simulink model "Autopilot_q_full_5may_new"  (R2020a)
settings: Solver=ode4  StartTime=0.0  StopTime=300  FixedStep=0.01  RelTol=1e-3
undefined symbols (not defined in the file or in its folder): Aero_cofficients, Atmosphere_pert, Atmospheric_model, Counter_sensor_model, Earth, error_global, flags_global, Guidance_Flags_global, INT_global, param_guidance, Payload_data, Plane_state_mode_finish_catcher_ftr_mode, Plane_state_mode_finish_catcher_fw_mode, Plane_state_mode_finish_catcher_q_mode, Plane_state_mode_finish_catcher_rtr_mode, Plane_state_store, propulsion_model, propulsion_model_int, Structural_data, Thrust_data_store, time_global, WGS84, Wind_data, Wind_model_int, Wind_pert_factor
libraries: simulink x33, aerolibactuator x15, cstblocks x3, aerolibatmos2 x2, aerolibfltsims x1, aerolibtransform2 x1, shared6dof x1
(part 5 of 10)

== system Autopilot_q_full_5may_new/AUTOPILOT /Autopilot Transition mode/Forward transition/Roll controller ==
  a_y_d : Inport
  In2 : Inport  Port=2
  Aero_coffecients read3 : DataStoreRead  DataStoreName=Aero_cofficients  DataStoreElements=Aero_cofficients(:,:)
  Constant{6..11} (6 alike) : Constant
  Data Store Read : DataStoreRead  DataStoreName=Thrust_data_store  DataStoreElements=Thrust_data_store(:,:)
  Data Store Read1 : DataStoreRead  DataStoreName=Plane_state_store  DataStoreElements=Plane_state_store(:,:)
  Data Store Read13 : DataStoreRead  DataStoreName=propulsion_model  DataStoreElements=propulsion_model(:)
  Data Store Read15 : DataStoreRead  DataStoreName=Atmospheric_model
  Data Store Read2 : DataStoreRead  DataStoreName=Wind_data  DataStoreElements=Wind_data(:)
  Digital Clock : DigitalClock  SampleTime=0.01
  Gain{,1..3} (4 alike) : Gain  Gain=57.3
  MATLAB Function1 : MATLAB Function  TreatAsAtomicUnit=on
  MATLAB Function2 : MATLAB Function  TreatAsAtomicUnit=on
  PID Controller (2DOF) : simulink/Continuous/PID Controller (2DOF)  Controller=PID  Form=Parallel  TimeDomain=Discrete-time  UseExternalTs=off  SampleTime=0.01  IntegratorMethod=Forward Euler  FilterMethod=Forward Euler  ControllerParametersSource=internal  P=2  I=0  D=0  UseFilter=on  N=100  b=1  c=1  TunerSelectOption=Transfer Function Based (PID Tuner App)  InitialConditionSource=internal  InitialConditionForIntegrator=0  InitialConditionForFilter=0  DifferentiatorICPrevScaledInput=0  ExternalReset=none  TrackingMode=off  Kt=1  LimitOutput=off  UpperSaturationLimit=inf  LowerSaturationLimit=-inf  LinearizeAsGain=on  AntiWindupMode=none  Kb=1  POutMin=[]  POutMax=[]  IOutMin=[]  IOutMax=[]  DOutMin=[]  DOutMax=[]  NOutMin=[]  NOutMax=[]  bOutMin=[]  bOutMax=[]  cOutMin=[]  cOutMax=[]  SumOutMin=[]  SumOutMax=[]  SaturationOutMin=[]  SaturationOutMax=[]  PParamMin=[]  PParamMax=[]  IParamMin=[]  IParamMax=[]  DParamMin=[]  DParamMax=[]  NParamMin=[]  NParamMax=[]  bParamMin=[]  bParamMax=[]  cParamMin=[]  cParamMax=[]  KbParamMin=[]  KbParamMax=[]  KtParamMin=[]  KtParamMax=[]  KbOutMin=[]  KbOutMax=[]  KtOutMin=[]  KtOutMax=[]  IntegratorOutMin=[]  IntegratorOutMax=[]  FilterOutMin=[]  FilterOutMax=[]  SumI1OutMin=[]  SumI1OutMax=[]  SumI2OutMin=[]  SumI2OutMax=[]  SumI3OutMin=[]  SumI3OutMax=[]  SumI4OutMin=[]  SumI4OutMax=[]  SumDOutMin=[]  SumDOutMax=[]  Sum1OutMin=[]  Sum1OutMax=[]  Sum2OutMin=[]  Sum2OutMax=[]  Sum3OutMin=[]  Sum3OutMax=[]  DifferentiatorOutMin=[]  DifferentiatorOutMax=[]  FilterDiffOutCoefMin=[]  FilterDiffOutCoefMax=[]  ReciprocalOutMin=[]  ReciprocalOutMax=[]  SumDenOutMin=[]  SumDenOutMax=[]  SumNumOutMin=[]  SumNumOutMax=[]  DivideOutMin=[]  DivideOutMax=[]  UdiffTsProdOutMin=[]  UdiffTsProdOutMax=[]  NTsProdOutMin=[]  NTsProdOutMax=[]  UintegralTsProdOutMin=[]  UintegralTsProdOutMax=[]  UngainTsProdOutMin=[]  UngainTsProdOutMax=[]  IntegratorContinuousStateAttributes=''  IntegratorStateMustResolveToSignalObject=off  IntegratorRTWStateStorageClass=Auto  FilterContinuousStateAttributes=''  FilterStateMustResolveToSignalObject=off  FilterRTWStateStorageClass=Auto  ParallelPVariant=InternalParameters  IdealPVariant=Disabled  IVariant=InternalParameters  DVariant=InternalParameters  bVariant=InternalParameters  cVariant=InternalParameters  IntegratorVariant=Discrete  SatVariant=Disabled  AWVariant=Passthrough  PCopyVariant=Disabled  TRVariant=Disabled  FdbkBlocksVariant=Forward  IdealPFdbkVariant=Disabled  SatFdbkVariant=Disabled  DerivativeFilterVariant=ForwardEulerFilter  NVariant=InternalParameters  NCopyVariant=Disabled  FilterICVariant=InternalICsFilter  IntegratorICVariant=InternalICs  ExternalResetVariant=Disabled  TRSumVariant=Passthrough  SumFdbkVariant=Disabled  SumVariant=Sum_PID  TsampFilterVariant=InternalTs  TsampNgainVariant=Passthrough  TsampIntegralVariant=Passthrough
  PID Controller (2DOF)1 : simulink/Continuous/PID Controller (2DOF)  Controller=PID  Form=Parallel  TimeDomain=Discrete-time  UseExternalTs=off  SampleTime=0.01  IntegratorMethod=Forward Euler  FilterMethod=Forward Euler  ControllerParametersSource=internal  P=6  I=1.0  D=0  UseFilter=on  N=100  b=1  c=1  TunerSelectOption=Transfer Function Based (PID Tuner App)  InitialConditionSource=internal  InitialConditionForIntegrator=0  InitialConditionForFilter=0  DifferentiatorICPrevScaledInput=0  ExternalReset=none  TrackingMode=off  Kt=1  LimitOutput=off  UpperSaturationLimit=inf  LowerSaturationLimit=-inf  LinearizeAsGain=on  AntiWindupMode=none  Kb=1  POutMin=[]  POutMax=[]  IOutMin=[]  IOutMax=[]  DOutMin=[]  DOutMax=[]  NOutMin=[]  NOutMax=[]  bOutMin=[]  bOutMax=[]  cOutMin=[]  cOutMax=[]  SumOutMin=[]  SumOutMax=[]  SaturationOutMin=[]  SaturationOutMax=[]  PParamMin=[]  PParamMax=[]  IParamMin=[]  IParamMax=[]  DParamMin=[]  DParamMax=[]  NParamMin=[]  NParamMax=[]  bParamMin=[]  bParamMax=[]  cParamMin=[]  cParamMax=[]  KbParamMin=[]  KbParamMax=[]  KtParamMin=[]  KtParamMax=[]  KbOutMin=[]  KbOutMax=[]  KtOutMin=[]  KtOutMax=[]  IntegratorOutMin=[]  IntegratorOutMax=[]  FilterOutMin=[]  FilterOutMax=[]  SumI1OutMin=[]  SumI1OutMax=[]  SumI2OutMin=[]  SumI2OutMax=[]  SumI3OutMin=[]  SumI3OutMax=[]  SumI4OutMin=[]  SumI4OutMax=[]  SumDOutMin=[]  SumDOutMax=[]  Sum1OutMin=[]  Sum1OutMax=[]  Sum2OutMin=[]  Sum2OutMax=[]  Sum3OutMin=[]  Sum3OutMax=[]  DifferentiatorOutMin=[]  DifferentiatorOutMax=[]  FilterDiffOutCoefMin=[]  FilterDiffOutCoefMax=[]  ReciprocalOutMin=[]  ReciprocalOutMax=[]  SumDenOutMin=[]  SumDenOutMax=[]  SumNumOutMin=[]  SumNumOutMax=[]  DivideOutMin=[]  DivideOutMax=[]  UdiffTsProdOutMin=[]  UdiffTsProdOutMax=[]  NTsProdOutMin=[]  NTsProdOutMax=[]  UintegralTsProdOutMin=[]  UintegralTsProdOutMax=[]  UngainTsProdOutMin=[]  UngainTsProdOutMax=[]  IntegratorContinuousStateAttributes=''  IntegratorStateMustResolveToSignalObject=off  IntegratorRTWStateStorageClass=Auto  FilterContinuousStateAttributes=''  FilterStateMustResolveToSignalObject=off  FilterRTWStateStorageClass=Auto  ParallelPVariant=InternalParameters  IdealPVariant=Disabled  IVariant=InternalParameters  DVariant=InternalParameters  bVariant=InternalParameters  cVariant=InternalParameters  IntegratorVariant=Discrete  SatVariant=Disabled  AWVariant=Passthrough  PCopyVariant=Disabled  TRVariant=Disabled  FdbkBlocksVariant=Forward  IdealPFdbkVariant=Disabled  SatFdbkVariant=Disabled  DerivativeFilterVariant=ForwardEulerFilter  NVariant=InternalParameters  NCopyVariant=Disabled  FilterICVariant=InternalICsFilter  IntegratorICVariant=InternalICs  ExternalResetVariant=Disabled  TRSumVariant=Passthrough  SumFdbkVariant=Disabled  SumVariant=Sum_PID  TsampFilterVariant=InternalTs  TsampNgainVariant=Passthrough  TsampIntegralVariant=Passthrough
  Scope : Scope  NumInputPorts=2
  Scope1 : Scope  NumInputPorts=2
  Structure_data_read2 : DataStoreRead  DataStoreName=Structural_data  DataStoreElements=Structural_data(:,:)
  mass : DataStoreRead  DataStoreName=Structural_data  DataStoreElements=Structural_data(1,1)
  p : DataStoreRead  DataStoreName=Plane_state_store  DataStoreElements=Plane_state_store(1,4)
  p,q,r,phi,theta,psi : DataStoreRead  DataStoreName=Plane_state_store  DataStoreElements=Plane_state_store(1,4:9)
  phi : DataStoreRead  DataStoreName=Plane_state_store  DataStoreElements=Plane_state_store(1,7)
  p_dot_d : Outport  VectorParamsAs1DForOutWhenUnconnected=off
  wires:
  p/1 -> Gain3/1, PID Controller (2DOF)1/2
  phi/1 -> Gain1/1, PID Controller (2DOF)/2
  p,q,r,phi,theta,psi/1 -> MATLAB Function2/1(angular_state)
  MATLAB Function2/1(p_d) -> Gain2/1, PID Controller (2DOF)1/1
  PID Controller (2DOF)/1 -> MATLAB Function2/2(phi_dot_d)
  mass/1 -> MATLAB Function1/3(mass)
  Data Store Read/1 -> MATLAB Function1/2(Thrust)
  Aero_coffecients read3/1 -> MATLAB Function1/5(aero_data)
  Digital Clock/1 -> MATLAB Function1/1(t)
  Structure_data_read2/1 -> MATLAB Function1/6(structure_data)
  MATLAB Function1/1(phi_d) -> Gain/1, PID Controller (2DOF)/1
  PID Controller (2DOF)1/1 -> p_dot_d/1
  a_y_d/1 -> MATLAB Function1/4(a_y_d)
  Data Store Read1/1 -> MATLAB Function1/7(Plane_state)
  Gain/1 -> Scope/1
  Gain1/1 -> Scope/2
  Gain2/1 -> Scope1/1
  Gain3/1 -> Scope1/2
  Data Store Read2/1 -> MATLAB Function1/8(Wind_ned)
  In2/1 -> MATLAB Function1/9(stall_speed)
  Data Store Read13/1 -> MATLAB Function1/10(propulsion_data)
  Data Store Read15/1 -> MATLAB Function1/11(atmos_data)
  Constant6/1 -> MATLAB Function1/12(data2)
  Constant7/1 -> MATLAB Function1/13(data3)
  Constant8/1 -> MATLAB Function1/14(data4)
  Constant9/1 -> MATLAB Function1/15(data5)
  Constant10/1 -> MATLAB Function1/16(data6)
  Constant11/1 -> MATLAB Function1/17(data7)

== system Autopilot_q_full_5may_new/AUTOPILOT /Autopilot Transition mode/Forward transition/Trim setting ==
  aero 1 : Inport
  struct 1 : Inport  Port=2
  V_trim1 : Inport  Port=3
  Data Store Read11 : DataStoreRead  DataStoreName=propulsion_model  DataStoreElements=propulsion_model(:)
  Data Store Read14 : DataStoreRead  DataStoreName=Atmospheric_model
  MATLAB Function1 : MATLAB Function  TreatAsAtomicUnit=on
  alpha_trim1 : Outport  VectorParamsAs1DForOutWhenUnconnected=off
  beta_trim1 : Outport  Port=2  VectorParamsAs1DForOutWhenUnconnected=off
  delta_e_trim1 : Outport  Port=3  VectorParamsAs1DForOutWhenUnconnected=off
  delta_a_trim1 : Outport  Port=4  VectorParamsAs1DForOutWhenUnconnected=off
  delta_r_trim1 : Outport  Port=5  VectorParamsAs1DForOutWhenUnconnected=off
  Tx_trim1 : Outport  Port=6  VectorParamsAs1DForOutWhenUnconnected=off
  stall_speed1 : Outport  Port=7  VectorParamsAs1DForOutWhenUnconnected=off
  wires:
  Data Store Read14/1 -> MATLAB Function1/5(atmos_data)
  Data Store Read11/1 -> MATLAB Function1/4(propulsion_data)
  MATLAB Function1/6(Tx_trim) -> Tx_trim1/1
  MATLAB Function1/2(beta_trim) -> beta_trim1/1
  MATLAB Function1/5(delta_r_trim) -> delta_r_trim1/1
  aero 1/1 -> MATLAB Function1/1(aero_data)
  struct 1/1 -> MATLAB Function1/2(structure_data)
  MATLAB Function1/4(delta_a_trim) -> delta_a_trim1/1
  MATLAB Function1/3(delta_e_trim) -> delta_e_trim1/1
  V_trim1/1 -> MATLAB Function1/3(V_trim)
  MATLAB Function1/7(stall_speed) -> stall_speed1/1
  MATLAB Function1/1(alpha_trim) -> alpha_trim1/1

== system Autopilot_q_full_5may_new/AUTOPILOT /Autopilot Transition mode/Reverse transition/Heading Controller ==
  psi_d1 : Inport
  Demux1 : Demux  Outputs=2
  Digital Clock : DigitalClock  SampleTime=0.01
  Gain{,1..3} (4 alike) : Gain  Gain=57.3
  MATLAB Function : MATLAB Function  TreatAsAtomicUnit=on
  MATLAB Function5 : MATLAB Function  TreatAsAtomicUnit=on
  MATLAB Function6 : MATLAB Function  TreatAsAtomicUnit=on
  PID Controller : simulink/Continuous/PID Controller  Controller=PID  Form=Parallel  TimeDomain=Discrete-time  UseExternalTs=off  SampleTime=0.01  IntegratorMethod=Forward Euler  FilterMethod=Forward Euler  ControllerParametersSource=internal  P=0.66  I=0  D=0  UseFilter=on  N=100  TunerSelectOption=Transfer Function Based (PID Tuner App)  InitialConditionSource=internal  InitialConditionForIntegrator=0  InitialConditionForFilter=0  DifferentiatorICPrevScaledInput=0  ExternalReset=none  TrackingMode=off  Kt=1  LimitOutput=off  UpperSaturationLimit=inf  LowerSaturationLimit=-inf  LinearizeAsGain=on  AntiWindupMode=none  Kb=1  POutMin=[]  POutMax=[]  IOutMin=[]  IOutMax=[]  DOutMin=[]  DOutMax=[]  NOutMin=[]  NOutMax=[]  SumOutMin=[]  SumOutMax=[]  SaturationOutMin=[]  SaturationOutMax=[]  PParamMin=[]  PParamMax=[]  IParamMin=[]  IParamMax=[]  DParamMin=[]  DParamMax=[]  NParamMin=[]  NParamMax=[]  KbParamMin=[]  KbParamMax=[]  KtParamMin=[]  KtParamMax=[]  KbOutMin=[]  KbOutMax=[]  KtOutMin=[]  KtOutMax=[]  IntegratorOutMin=[]  IntegratorOutMax=[]  FilterOutMin=[]  FilterOutMax=[]  SumI1OutMin=[]  SumI1OutMax=[]  SumI2OutMin=[]  SumI2OutMax=[]  SumI3OutMin=[]  SumI3OutMax=[]  SumI4OutMin=[]  SumI4OutMax=[]  SumDOutMin=[]  SumDOutMax=[]  DifferentiatorOutMin=[]  DifferentiatorOutMax=[]  FilterDiffOutCoefMin=[]  FilterDiffOutCoefMax=[]  ReciprocalOutMin=[]  ReciprocalOutMax=[]  SumDenOutMin=[]  SumDenOutMax=[]  SumNumOutMin=[]  SumNumOutMax=[]  DivideOutMin=[]  DivideOutMax=[]  UdiffTsProdOutMin=[]  UdiffTsProdOutMax=[]  NTsProdOutMin=[]  NTsProdOutMax=[]  UintegralTsProdOutMin=[]  UintegralTsProdOutMax=[]  UngainTsProdOutMin=[]  UngainTsProdOutMax=[]  IntegratorContinuousStateAttributes=''  IntegratorStateMustResolveToSignalObject=off  IntegratorRTWStateStorageClass=Auto  FilterContinuousStateAttributes=''  FilterStateMustResolveToSignalObject=off  FilterRTWStateStorageClass=Auto  ParallelPVariant=InternalParameters  IdealPVariant=Disabled  IVariant=InternalParameters  DVariant=InternalParameters  IntegratorVariant=Discrete  SatVariant=Disabled  AWVariant=Passthrough  PCopyVariant=Disabled  TRVariant=Disabled  FdbkBlocksVariant=Forward  IdealPFdbkVariant=Disabled  SatFdbkVariant=Disabled  DerivativeFilterVariant=ForwardEulerFilter  NVariant=InternalParameters  NCopyVariant=Disabled  FilterICVariant=InternalICsFilter  IntegratorICVariant=InternalICs  ExternalResetVariant=Disabled  TRSumVariant=Passthrough  SumFdbkVariant=Disabled  SumVariant=Sum_PID  TsampFilterVariant=InternalTs  TsampNgainVariant=Passthrough  TsampIntegralVariant=Passthrough
  PID Controller (2DOF)5 : simulink/Continuous/PID Controller (2DOF)  Controller=PID  Form=Parallel  TimeDomain=Discrete-time  UseExternalTs=off  SampleTime=0.01  IntegratorMethod=Forward Euler  FilterMethod=Forward Euler  ControllerParametersSource=internal  P=2.0  I=0.5  D=0  UseFilter=on  N=100  b=1  c=1  TunerSelectOption=Transfer Function Based (PID Tuner App)  InitialConditionSource=internal  InitialConditionForIntegrator=0  InitialConditionForFilter=0  DifferentiatorICPrevScaledInput=0  ExternalReset=none  TrackingMode=off  Kt=1  LimitOutput=off  UpperSaturationLimit=inf  LowerSaturationLimit=-inf  LinearizeAsGain=on  AntiWindupMode=none  Kb=1  POutMin=[]  POutMax=[]  IOutMin=[]  IOutMax=[]  DOutMin=[]  DOutMax=[]  NOutMin=[]  NOutMax=[]  bOutMin=[]  bOutMax=[]  cOutMin=[]  cOutMax=[]  SumOutMin=[]  SumOutMax=[]  SaturationOutMin=[]  SaturationOutMax=[]  PParamMin=[]  PParamMax=[]  IParamMin=[]  IParamMax=[]  DParamMin=[]  DParamMax=[]  NParamMin=[]  NParamMax=[]  bParamMin=[]  bParamMax=[]  cParamMin=[]  cParamMax=[]  KbParamMin=[]  KbParamMax=[]  KtParamMin=[]  KtParamMax=[]  KbOutMin=[]  KbOutMax=[]  KtOutMin=[]  KtOutMax=[]  IntegratorOutMin=[]  IntegratorOutMax=[]  FilterOutMin=[]  FilterOutMax=[]  SumI1OutMin=[]  SumI1OutMax=[]  SumI2OutMin=[]  SumI2OutMax=[]  SumI3OutMin=[]  SumI3OutMax=[]  SumI4OutMin=[]  SumI4OutMax=[]  SumDOutMin=[]  SumDOutMax=[]  Sum1OutMin=[]  Sum1OutMax=[]  Sum2OutMin=[]  Sum2OutMax=[]  Sum3OutMin=[]  Sum3OutMax=[]  DifferentiatorOutMin=[]  DifferentiatorOutMax=[]  FilterDiffOutCoefMin=[]  FilterDiffOutCoefMax=[]  ReciprocalOutMin=[]  ReciprocalOutMax=[]  SumDenOutMin=[]  SumDenOutMax=[]  SumNumOutMin=[]  SumNumOutMax=[]  DivideOutMin=[]  DivideOutMax=[]  UdiffTsProdOutMin=[]  UdiffTsProdOutMax=[]  NTsProdOutMin=[]  NTsProdOutMax=[]  UintegralTsProdOutMin=[]  UintegralTsProdOutMax=[]  UngainTsProdOutMin=[]  UngainTsProdOutMax=[]  IntegratorContinuousStateAttributes=''  IntegratorStateMustResolveToSignalObject=off  IntegratorRTWStateStorageClass=Auto  FilterContinuousStateAttributes=''  FilterStateMustResolveToSignalObject=off  FilterRTWStateStorageClass=Auto  ParallelPVariant=InternalParameters  IdealPVariant=Disabled  IVariant=InternalParameters  DVariant=InternalParameters  bVariant=InternalParameters  cVariant=InternalParameters  IntegratorVariant=Discrete  SatVariant=Disabled  AWVariant=Passthrough  PCopyVariant=Disabled  TRVariant=Disabled  FdbkBlocksVariant=Forward  IdealPFdbkVariant=Disabled  SatFdbkVariant=Disabled  DerivativeFilterVariant=ForwardEulerFilter  NVariant=InternalParameters  NCopyVariant=Disabled  FilterICVariant=InternalICsFilter  IntegratorICVariant=InternalICs  ExternalResetVariant=Disabled  TRSumVariant=Passthrough  SumFdbkVariant=Disabled  SumVariant=Sum_PID  TsampFilterVariant=InternalTs  TsampNgainVariant=Passthrough  TsampIntegralVariant=Passthrough
  Scope : Scope  NumInputPorts=2
  Scope1 : Scope  NumInputPorts=2
  p,q,r,phi,theta,psi : DataStoreRead  DataStoreName=Plane_state_store  DataStoreElements=Plane_state_store(1,4:9)
  psi : DataStoreRead  DataStoreName=Plane_state_store  DataStoreElements=Plane_state_store(1,9)
  r : DataStoreRead  DataStoreName=Plane_state_store  DataStoreElements=Plane_state_store(1,6)
  u,v : DataStoreRead  DataStoreName=Plane_state_store  DataStoreElements=Plane_state_store(1,1:2)
  r_dot_d : Outport  VectorParamsAs1DForOutWhenUnconnected=off
  wires:
  u,v/1 -> Demux1/1
  MATLAB Function/1(psi_error) -> PID Controller/1
  Demux1/2 -> MATLAB Function5/3(v)
  r/1 -> Gain3/1, PID Controller (2DOF)5/2
  psi/1 -> MATLAB Function/2(psi), Gain1/1
  p,q,r,phi,theta,psi/1 -> MATLAB Function6/1(angular_state)
  MATLAB Function5/1(psi_d) -> Gain/1, MATLAB Function/1(psi_d)
  PID Controller/1 -> MATLAB Function6/2(psi_dot_d)
  MATLAB Function6/1(r_d) -> PID Controller (2DOF)5/1, Gain2/1
  Demux1/1 -> MATLAB Function5/2(u)
  PID Controller (2DOF)5/1 -> r_dot_d/1
  Digital Clock/1 -> MATLAB Function5/1(t)
  psi_d1/1 -> MATLAB Function5/4("psi_d ")
  Gain/1 -> Scope/1
  Gain1/1 -> Scope/2
  Gain2/1 -> Scope1/1
  Gain3/1 -> Scope1/2

== system Autopilot_q_full_5may_new/AUTOPILOT /Autopilot Transition mode/Reverse transition/Pitch Controller ==
  a_x_d : Inport
  Speed : Inport  Port=2
  acc_d : Inport  Port=3
  alpha_trim : Inport  Port=4
  Stall_speed : Inport  Port=5
  Data Store Read1 : DataStoreRead  DataStoreName=Plane_state_store  DataStoreElements=Plane_state_store(:,:)
  Digital Clock : DigitalClock  SampleTime=0.01
  If : If  NumInputs=2  IfExpression=u1 < u2
  MATLAB Function : MATLAB Function  TreatAsAtomicUnit=on
  MATLAB Function3 : MATLAB Function  TreatAsAtomicUnit=on
  MATLAB Function4 : MATLAB Function  TreatAsAtomicUnit=on
  PID Controller (2DOF)3 : simulink/Continuous/PID Controller (2DOF)  Controller=PID  Form=Parallel  TimeDomain=Discrete-time  UseExternalTs=off  SampleTime=0.01  IntegratorMethod=Forward Euler  FilterMethod=Forward Euler  ControllerParametersSource=internal  P=6.0  I=2.0  D=0  UseFilter=on  N=100  b=1  c=1  TunerSelectOption=Transfer Function Based (PID Tuner App)  InitialConditionSource=internal  InitialConditionForIntegrator=0  InitialConditionForFilter=0  DifferentiatorICPrevScaledInput=0  ExternalReset=none  TrackingMode=off  Kt=1  LimitOutput=off  UpperSaturationLimit=inf  LowerSaturationLimit=-inf  LinearizeAsGain=on  AntiWindupMode=none  Kb=1  POutMin=[]  POutMax=[]  IOutMin=[]  IOutMax=[]  DOutMin=[]  DOutMax=[]  NOutMin=[]  NOutMax=[]  bOutMin=[]  bOutMax=[]  cOutMin=[]  cOutMax=[]  SumOutMin=[]  SumOutMax=[]  SaturationOutMin=[]  SaturationOutMax=[]  PParamMin=[]  PParamMax=[]  IParamMin=[]  IParamMax=[]  DParamMin=[]  DParamMax=[]  NParamMin=[]  NParamMax=[]  bParamMin=[]  bParamMax=[]  cParamMin=[]  cParamMax=[]  KbParamMin=[]  KbParamMax=[]  KtParamMin=[]  KtParamMax=[]  KbOutMin=[]  KbOutMax=[]  KtOutMin=[]  KtOutMax=[]  IntegratorOutMin=[]  IntegratorOutMax=[]  FilterOutMin=[]  FilterOutMax=[]  SumI1OutMin=[]  SumI1OutMax=[]  SumI2OutMin=[]  SumI2OutMax=[]  SumI3OutMin=[]  SumI3OutMax=[]  SumI4OutMin=[]  SumI4OutMax=[]  SumDOutMin=[]  SumDOutMax=[]  Sum1OutMin=[]  Sum1OutMax=[]  Sum2OutMin=[]  Sum2OutMax=[]  Sum3OutMin=[]  Sum3OutMax=[]  DifferentiatorOutMin=[]  DifferentiatorOutMax=[]  FilterDiffOutCoefMin=[]  FilterDiffOutCoefMax=[]  ReciprocalOutMin=[]  ReciprocalOutMax=[]  SumDenOutMin=[]  SumDenOutMax=[]  SumNumOutMin=[]  SumNumOutMax=[]  DivideOutMin=[]  DivideOutMax=[]  UdiffTsProdOutMin=[]  UdiffTsProdOutMax=[]  NTsProdOutMin=[]  NTsProdOutMax=[]  UintegralTsProdOutMin=[]  UintegralTsProdOutMax=[]  UngainTsProdOutMin=[]  UngainTsProdOutMax=[]  IntegratorContinuousStateAttributes=''  IntegratorStateMustResolveToSignalObject=off  IntegratorRTWStateStorageClass=Auto  FilterContinuousStateAttributes=''  FilterStateMustResolveToSignalObject=off  FilterRTWStateStorageClass=Auto  ParallelPVariant=InternalParameters  IdealPVariant=Disabled  IVariant=InternalParameters  DVariant=InternalParameters  bVariant=InternalParameters  cVariant=InternalParameters  IntegratorVariant=Discrete  SatVariant=Disabled  AWVariant=Passthrough  PCopyVariant=Disabled  TRVariant=Disabled  FdbkBlocksVariant=Forward  IdealPFdbkVariant=Disabled  SatFdbkVariant=Disabled  DerivativeFilterVariant=ForwardEulerFilter  NVariant=InternalParameters  NCopyVariant=Disabled  FilterICVariant=InternalICsFilter  IntegratorICVariant=InternalICs  ExternalResetVariant=Disabled  TRSumVariant=Passthrough  SumFdbkVariant=Disabled  SumVariant=Sum_PID  TsampFilterVariant=InternalTs  TsampNgainVariant=Passthrough  TsampIntegralVariant=Passthrough
  Switch : Switch  Criteria=u2 ~= 0  Threshold=7/57.3
  alpha controller : Subsystem  TreatAsAtomicUnit=on
  p,q,r,phi,theta,psi : DataStoreRead  DataStoreName=Plane_state_store  DataStoreElements=Plane_state_store(1,4:9)
  "q " : DataStoreRead  DataStoreName=Plane_state_store  DataStoreElements=Plane_state_store(1,5)
  theta controller : Subsystem  TreatAsAtomicUnit=on
  q_dot_d : Outport  VectorParamsAs1DForOutWhenUnconnected=off
  wires:
  Speed/1 -> MATLAB Function/1(u1), If/1
  alpha controller/1(Output) -> MATLAB Function3/2(alpha_dot_d)
  Stall_speed/1 -> MATLAB Function/2(u2), If/2
  theta controller/1(theta_dot) -> MATLAB Function4/1(theta_dot_d)
  Switch/1 -> PID Controller (2DOF)3/1
  Digital Clock/1 -> theta controller/1(time)
  MATLAB Function4/1(q_d) -> Switch/1
  "q "/1 -> PID Controller (2DOF)3/2
  MATLAB Function3/1(q_d) -> Switch/3
  MATLAB Function/1(y) -> Switch/2
  Data Store Read1/1 -> alpha controller/2(Plane_state)
  acc_d/1 -> alpha controller/1(acc_d)
  alpha_trim/1 -> theta controller/3(alpha_trim)
  PID Controller (2DOF)3/1 -> q_dot_d/1
  a_x_d/1 -> theta controller/2(a_x_d)
  If/2 -> alpha controller/Action
  If/1 -> theta controller/Action
  p,q,r,phi,theta,psi/1 -> MATLAB Function3/1(angular_state), MATLAB Function4/2(angular_state)

== system Autopilot_q_full_5may_new/AUTOPILOT /Autopilot Transition mode/Reverse transition/Roll controller ==
  a_y_d : Inport
  Stall_speed : Inport  Port=2
  Aero_coffecients read3 : DataStoreRead  DataStoreName=Aero_cofficients  DataStoreElements=Aero_cofficients(:,:)
  Constant{6..11} (6 alike) : Constant
  Data Store Read : DataStoreRead  DataStoreName=Thrust_data_store  DataStoreElements=Thrust_data_store(:,:)
  Data Store Read1 : DataStoreRead  DataStoreName=Plane_state_store  DataStoreElements=Plane_state_store(:,:)
  Data Store Read13 : DataStoreRead  DataStoreName=propulsion_model  DataStoreElements=propulsion_model(:)
  Data Store Read15 : DataStoreRead  DataStoreName=Atmospheric_model
  Data Store Read2 : DataStoreRead  DataStoreName=Wind_data  DataStoreElements=Wind_data(:)
  Digital Clock : DigitalClock  SampleTime=0.01
  Gain{,1..3} (4 alike) : Gain  Gain=57.3
  MATLAB Function1 : MATLAB Function  TreatAsAtomicUnit=on
  MATLAB Function2 : MATLAB Function  TreatAsAtomicUnit=on
  PID Controller (2DOF) : simulink/Continuous/PID Controller (2DOF)  Controller=PID  Form=Parallel  TimeDomain=Discrete-time  UseExternalTs=off  SampleTime=0.01  IntegratorMethod=Forward Euler  FilterMethod=Forward Euler  ControllerParametersSource=internal  P=2  I=0  D=0  UseFilter=on  N=100  b=1  c=1  TunerSelectOption=Transfer Function Based (PID Tuner App)  InitialConditionSource=internal  InitialConditionForIntegrator=0  InitialConditionForFilter=0  DifferentiatorICPrevScaledInput=0  ExternalReset=none  TrackingMode=off  Kt=1  LimitOutput=off  UpperSaturationLimit=inf  LowerSaturationLimit=-inf  LinearizeAsGain=on  AntiWindupMode=none  Kb=1  POutMin=[]  POutMax=[]  IOutMin=[]  IOutMax=[]  DOutMin=[]  DOutMax=[]  NOutMin=[]  NOutMax=[]  bOutMin=[]  bOutMax=[]  cOutMin=[]  cOutMax=[]  SumOutMin=[]  SumOutMax=[]  SaturationOutMin=[]  SaturationOutMax=[]  PParamMin=[]  PParamMax=[]  IParamMin=[]  IParamMax=[]  DParamMin=[]  DParamMax=[]  NParamMin=[]  NParamMax=[]  bParamMin=[]  bParamMax=[]  cParamMin=[]  cParamMax=[]  KbParamMin=[]  KbParamMax=[]  KtParamMin=[]  KtParamMax=[]  KbOutMin=[]  KbOutMax=[]  KtOutMin=[]  KtOutMax=[]  IntegratorOutMin=[]  IntegratorOutMax=[]  FilterOutMin=[]  FilterOutMax=[]  SumI1OutMin=[]  SumI1OutMax=[]  SumI2OutMin=[]  SumI2OutMax=[]  SumI3OutMin=[]  SumI3OutMax=[]  SumI4OutMin=[]  SumI4OutMax=[]  SumDOutMin=[]  SumDOutMax=[]  Sum1OutMin=[]  Sum1OutMax=[]  Sum2OutMin=[]  Sum2OutMax=[]  Sum3OutMin=[]  Sum3OutMax=[]  DifferentiatorOutMin=[]  DifferentiatorOutMax=[]  FilterDiffOutCoefMin=[]  FilterDiffOutCoefMax=[]  ReciprocalOutMin=[]  ReciprocalOutMax=[]  SumDenOutMin=[]  SumDenOutMax=[]  SumNumOutMin=[]  SumNumOutMax=[]  DivideOutMin=[]  DivideOutMax=[]  UdiffTsProdOutMin=[]  UdiffTsProdOutMax=[]  NTsProdOutMin=[]  NTsProdOutMax=[]  UintegralTsProdOutMin=[]  UintegralTsProdOutMax=[]  UngainTsProdOutMin=[]  UngainTsProdOutMax=[]  IntegratorContinuousStateAttributes=''  IntegratorStateMustResolveToSignalObject=off  IntegratorRTWStateStorageClass=Auto  FilterContinuousStateAttributes=''  FilterStateMustResolveToSignalObject=off  FilterRTWStateStorageClass=Auto  ParallelPVariant=InternalParameters  IdealPVariant=Disabled  IVariant=InternalParameters  DVariant=InternalParameters  bVariant=InternalParameters  cVariant=InternalParameters  IntegratorVariant=Discrete  SatVariant=Disabled  AWVariant=Passthrough  PCopyVariant=Disabled  TRVariant=Disabled  FdbkBlocksVariant=Forward  IdealPFdbkVariant=Disabled  SatFdbkVariant=Disabled  DerivativeFilterVariant=ForwardEulerFilter  NVariant=InternalParameters  NCopyVariant=Disabled  FilterICVariant=InternalICsFilter  IntegratorICVariant=InternalICs  ExternalResetVariant=Disabled  TRSumVariant=Passthrough  SumFdbkVariant=Disabled  SumVariant=Sum_PID  TsampFilterVariant=InternalTs  TsampNgainVariant=Passthrough  TsampIntegralVariant=Passthrough
  PID Controller (2DOF)1 : simulink/Continuous/PID Controller (2DOF)  Controller=PID  Form=Parallel  TimeDomain=Discrete-time  UseExternalTs=off  SampleTime=0.01  IntegratorMethod=Forward Euler  FilterMethod=Forward Euler  ControllerParametersSource=internal  P=6  I=2.0  D=0  UseFilter=on  N=100  b=1  c=1  TunerSelectOption=Transfer Function Based (PID Tuner App)  InitialConditionSource=internal  InitialConditionForIntegrator=0  InitialConditionForFilter=0  DifferentiatorICPrevScaledInput=0  ExternalReset=none  TrackingMode=off  Kt=1  LimitOutput=off  UpperSaturationLimit=inf  LowerSaturationLimit=-inf  LinearizeAsGain=on  AntiWindupMode=none  Kb=1  POutMin=[]  POutMax=[]  IOutMin=[]  IOutMax=[]  DOutMin=[]  DOutMax=[]  NOutMin=[]  NOutMax=[]  bOutMin=[]  bOutMax=[]  cOutMin=[]  cOutMax=[]  SumOutMin=[]  SumOutMax=[]  SaturationOutMin=[]  SaturationOutMax=[]  PParamMin=[]  PParamMax=[]  IParamMin=[]  IParamMax=[]  DParamMin=[]  DParamMax=[]  NParamMin=[]  NParamMax=[]  bParamMin=[]  bParamMax=[]  cParamMin=[]  cParamMax=[]  KbParamMin=[]  KbParamMax=[]  KtParamMin=[]  KtParamMax=[]  KbOutMin=[]  KbOutMax=[]  KtOutMin=[]  KtOutMax=[]  IntegratorOutMin=[]  IntegratorOutMax=[]  FilterOutMin=[]  FilterOutMax=[]  SumI1OutMin=[]  SumI1OutMax=[]  SumI2OutMin=[]  SumI2OutMax=[]  SumI3OutMin=[]  SumI3OutMax=[]  SumI4OutMin=[]  SumI4OutMax=[]  SumDOutMin=[]  SumDOutMax=[]  Sum1OutMin=[]  Sum1OutMax=[]  Sum2OutMin=[]  Sum2OutMax=[]  Sum3OutMin=[]  Sum3OutMax=[]  DifferentiatorOutMin=[]  DifferentiatorOutMax=[]  FilterDiffOutCoefMin=[]  FilterDiffOutCoefMax=[]  ReciprocalOutMin=[]  ReciprocalOutMax=[]  SumDenOutMin=[]  SumDenOutMax=[]  SumNumOutMin=[]  SumNumOutMax=[]  DivideOutMin=[]  DivideOutMax=[]  UdiffTsProdOutMin=[]  UdiffTsProdOutMax=[]  NTsProdOutMin=[]  NTsProdOutMax=[]  UintegralTsProdOutMin=[]  UintegralTsProdOutMax=[]  UngainTsProdOutMin=[]  UngainTsProdOutMax=[]  IntegratorContinuousStateAttributes=''  IntegratorStateMustResolveToSignalObject=off  IntegratorRTWStateStorageClass=Auto  FilterContinuousStateAttributes=''  FilterStateMustResolveToSignalObject=off  FilterRTWStateStorageClass=Auto  ParallelPVariant=InternalParameters  IdealPVariant=Disabled  IVariant=InternalParameters  DVariant=InternalParameters  bVariant=InternalParameters  cVariant=InternalParameters  IntegratorVariant=Discrete  SatVariant=Disabled  AWVariant=Passthrough  PCopyVariant=Disabled  TRVariant=Disabled  FdbkBlocksVariant=Forward  IdealPFdbkVariant=Disabled  SatFdbkVariant=Disabled  DerivativeFilterVariant=ForwardEulerFilter  NVariant=InternalParameters  NCopyVariant=Disabled  FilterICVariant=InternalICsFilter  IntegratorICVariant=InternalICs  ExternalResetVariant=Disabled  TRSumVariant=Passthrough  SumFdbkVariant=Disabled  SumVariant=Sum_PID  TsampFilterVariant=InternalTs  TsampNgainVariant=Passthrough  TsampIntegralVariant=Passthrough
  Scope : Scope  NumInputPorts=2
  Scope1 : Scope  NumInputPorts=2
  Structure_data_read2 : DataStoreRead  DataStoreName=Structural_data  DataStoreElements=Structural_data(:,:)
  ang_st : DataStoreRead  DataStoreName=Plane_state_store  DataStoreElements=Plane_state_store(1,4:9)
  mass : DataStoreRead  DataStoreName=Structural_data  DataStoreElements=Structural_data(1,1)
  p : DataStoreRead  DataStoreName=Plane_state_store  DataStoreElements=Plane_state_store(1,4)
  phi : DataStoreRead  DataStoreName=Plane_state_store  DataStoreElements=Plane_state_store(1,7)
  p_dot_d : Outport  VectorParamsAs1DForOutWhenUnconnected=off
  wires:
  p/1 -> Gain3/1, PID Controller (2DOF)1/2
  phi/1 -> Gain1/1, PID Controller (2DOF)/2
  ang_st/1 -> MATLAB Function2/1(angular_state)
  MATLAB Function2/1(p_d) -> Gain2/1, PID Controller (2DOF)1/1
  PID Controller (2DOF)/1 -> MATLAB Function2/2(phi_dot_d)
  mass/1 -> MATLAB Function1/3(mass)
  Data Store Read/1 -> MATLAB Function1/2(Thrust)
  Aero_coffecients read3/1 -> MATLAB Function1/5(aero_data)
  Digital Clock/1 -> MATLAB Function1/1(t)
  Structure_data_read2/1 -> MATLAB Function1/6(structure_data)
  MATLAB Function1/1(phi_d) -> Gain/1, PID Controller (2DOF)/1
  PID Controller (2DOF)1/1 -> p_dot_d/1
  a_y_d/1 -> MATLAB Function1/4(a_y_d)
  Data Store Read1/1 -> MATLAB Function1/7(Plane_state)
  Stall_speed/1 -> MATLAB Function1/8(Stall_speed)
  Gain/1 -> Scope/1
  Gain1/1 -> Scope/2
  Gain2/1 -> Scope1/1
  Gain3/1 -> Scope1/2
  Data Store Read2/1 -> MATLAB Function1/9(Wind_ned)
  Data Store Read13/1 -> MATLAB Function1/10(propulsion_data)
  Data Store Read15/1 -> MATLAB Function1/11(atmos_data)
  Constant6/1 -> MATLAB Function1/12(data2)
  Constant7/1 -> MATLAB Function1/13(data3)
  Constant8/1 -> MATLAB Function1/14(data4)
  Constant9/1 -> MATLAB Function1/15(data5)
  Constant10/1 -> MATLAB Function1/16(data6)
  Constant11/1 -> MATLAB Function1/17(data7)

== system Autopilot_q_full_5may_new/AUTOPILOT /Autopilot Transition mode/Reverse transition/Trim setting ==
  "aero " : Inport
  "struct " : Inport  Port=2
  V_trim : Inport  Port=3
  Data Store Read11 : DataStoreRead  DataStoreName=propulsion_model  DataStoreElements=propulsion_model(:)
  Data Store Read14 : DataStoreRead  DataStoreName=Atmospheric_model
  MATLAB Function : MATLAB Function  TreatAsAtomicUnit=on
  alpha_trim : Outport  VectorParamsAs1DForOutWhenUnconnected=off
  beta_trim : Outport  Port=2  VectorParamsAs1DForOutWhenUnconnected=off
  delta_e_trim : Outport  Port=3  VectorParamsAs1DForOutWhenUnconnected=off
  delta_a_trim : Outport  Port=4  VectorParamsAs1DForOutWhenUnconnected=off
  delta_r_trim : Outport  Port=5  VectorParamsAs1DForOutWhenUnconnected=off
  Tx_trim : Outport  Port=6  VectorParamsAs1DForOutWhenUnconnected=off
  stall_speed : Outport  Port=7  VectorParamsAs1DForOutWhenUnconnected=off
  wires:
  "aero "/1 -> MATLAB Function/1(aero_data)
  "struct "/1 -> MATLAB Function/2(structure_data)
  V_trim/1 -> MATLAB Function/3(V_trim)
  MATLAB Function/1(alpha_trim) -> alpha_trim/1
  MATLAB Function/2(beta_trim) -> beta_trim/1
  MATLAB Function/3(delta_e_trim) -> delta_e_trim/1
  MATLAB Function/4(delta_a_trim) -> delta_a_trim/1
  MATLAB Function/5(delta_r_trim) -> delta_r_trim/1
  MATLAB Function/6(Tx_trim) -> Tx_trim/1
  MATLAB Function/7(stall_speed) -> stall_speed/1
  Data Store Read11/1 -> MATLAB Function/4(propulsion_data)
  Data Store Read14/1 -> MATLAB Function/5(atmos_data)

== system Autopilot_q_full_5may_new/INITIALISE_PARAMS/If Action Subsystem/Aero_data_perturbation/Subsystem1 ==
  In1 : Inport
  Constant : Constant  Value=0
  Subsystem : Subsystem
  Switch : Switch  Criteria=u2 > Threshold
  Out1 : Outport  VectorParamsAs1DForOutWhenUnconnected=off
  wires:
  Subsystem/1(Out1) -> Switch/3
  In1/1 -> Switch/1
  Switch/1 -> Out1/1
  Constant/1 -> Switch/2

== system Autopilot_q_full_5may_new/INITIALISE_PARAMS/If Action Subsystem/Aero_data_perturbation/Subsystem2 ==
  In1 : Inport
  Constant : Constant  Value=0
  Subsystem : Subsystem
  Switch : Switch  Criteria=u2 > Threshold
  Out1 : Outport  VectorParamsAs1DForOutWhenUnconnected=off
  wires:
  Constant/1 -> Switch/2
  Switch/1 -> Out1/1
  In1/1 -> Switch/1
  Subsystem/1(Out1) -> Switch/3

== system Autopilot_q_full_5may_new/INITIALISE_PARAMS/If Action Subsystem/Aero_data_perturbation/Subsystem3 ==
  In1 : Inport
  Constant : Constant  Value=0
  Subsystem : Subsystem
  Switch : Switch  Criteria=u2 > Threshold
  Out1 : Outport  VectorParamsAs1DForOutWhenUnconnected=off
  wires:
  Subsystem/1(Out1) -> Switch/3
  In1/1 -> Switch/1
  Switch/1 -> Out1/1
  Constant/1 -> Switch/2

== system Autopilot_q_full_5may_new/INITIALISE_PARAMS/If Action Subsystem/Aero_data_perturbation/Subsystem4 ==
  In1 : Inport
  Constant : Constant  Value=0
  Subsystem : Subsystem
  Switch : Switch  Criteria=u2 > Threshold
  Out1 : Outport  VectorParamsAs1DForOutWhenUnconnected=off
  wires:
  Constant/1 -> Switch/2
  Switch/1 -> Out1/1
  In1/1 -> Switch/1
  Subsystem/1(Out1) -> Switch/3

== system Autopilot_q_full_5may_new/INITIALISE_PARAMS/If Action Subsystem/Aero_data_perturbation/Subsystem5 ==
  In1 : Inport
  Constant : Constant  Value=0
  Subsystem : Subsystem
  Switch : Switch  Criteria=u2 > Threshold
  Out1 : Outport  VectorParamsAs1DForOutWhenUnconnected=off
  wires:
  Subsystem/1(Out1) -> Switch/3
  In1/1 -> Switch/1
  Switch/1 -> Out1/1
  Constant/1 -> Switch/2

== system Autopilot_q_full_5may_new/INITIALISE_PARAMS/If Action Subsystem/Aero_data_perturbation/Subsystem6 ==
  In1 : Inport
  Constant : Constant  Value=0
  Subsystem : Subsystem
  Switch : Switch  Criteria=u2 > Threshold
  Out1 : Outport  VectorParamsAs1DForOutWhenUnconnected=off
  wires:
  Constant/1 -> Switch/2
  Switch/1 -> Out1/1
  In1/1 -> Switch/1
  Subsystem/1(Out1) -> Switch/3

== system Autopilot_q_full_5may_new/INITIALISE_PARAMS/If Action Subsystem/Atmosphere_pert/Subsystem1 ==
  In1 : Inport
  Constant : Constant  Value=0
  Subsystem : Subsystem
  Switch : Switch  Criteria=u2 > Threshold
  Out1 : Outport  VectorParamsAs1DForOutWhenUnconnected=off
  wires:
  Subsystem/1(Out1) -> Switch/3
  In1/1 -> Switch/1
  Switch/1 -> Out1/1
  Constant/1 -> Switch/2

== system Autopilot_q_full_5may_new/INITIALISE_PARAMS/If Action Subsystem/Propulsion_data_pert/Subsystem1 ==
  In1 : Inport
  Constant : Constant  Value=0
  Subsystem : Subsystem
  Switch : Switch  Criteria=u2 > Threshold
  Out1 : Outport  VectorParamsAs1DForOutWhenUnconnected=off
  wires:
  Subsystem/1(Out1) -> Switch/3
  In1/1 -> Switch/1
  Switch/1 -> Out1/1
  Constant/1 -> Switch/2

== system Autopilot_q_full_5may_new/INITIALISE_PARAMS/If Action Subsystem/Propulsion_data_pert/Subsystem2 ==
  In1 : Inport
  Constant : Constant  Value=0
  Subsystem : Subsystem
  Switch : Switch  Criteria=u2 > Threshold
  Out1 : Outport  VectorParamsAs1DForOutWhenUnconnected=off
  wires:
  Subsystem/1(Out1) -> Switch/3
  In1/1 -> Switch/1
  Switch/1 -> Out1/1
  Constant/1 -> Switch/2

== system Autopilot_q_full_5may_new/INITIALISE_PARAMS/If Action Subsystem/Structure_data_pert/Subsystem1 ==
  In1 : Inport
  Constant : Constant  Value=0
  Subsystem : Subsystem
  Switch : Switch  Criteria=u2 > Threshold
  Out1 : Outport  VectorParamsAs1DForOutWhenUnconnected=off
  wires:
  Constant/1 -> Switch/2
  Switch/1 -> Out1/1
  In1/1 -> Switch/1
  Subsystem/1(Out1) -> Switch/3

== system Autopilot_q_full_5may_new/INITIALISE_PARAMS/If Action Subsystem/Structure_data_pert/Subsystem2 ==
  In1 : Inport
  Constant : Constant  Value=0
  Subsystem : Subsystem
  Switch : Switch  Criteria=u2 > Threshold
  Out1 : Outport  VectorParamsAs1DForOutWhenUnconnected=off
  wires:
  Subsystem/1(Out1) -> Switch/3
  In1/1 -> Switch/1
  Switch/1 -> Out1/1
  Constant/1 -> Switch/2

== system Autopilot_q_full_5may_new/INITIALISE_PARAMS/If Action Subsystem/Structure_data_pert/Subsystem3 ==
  In1 : Inport
  Constant : Constant  Value=0
  Subsystem : Subsystem
  Switch : Switch  Criteria=u2 > Threshold
  Out1 : Outport  VectorParamsAs1DForOutWhenUnconnected=off
  wires:
  Constant/1 -> Switch/2
  Switch/1 -> Out1/1
  In1/1 -> Switch/1
  Subsystem/1(Out1) -> Switch/3

== system Autopilot_q_full_5may_new/INITIALISE_PARAMS/If Action Subsystem/Structure_data_pert/Subsystem4 ==
  In1 : Inport
  Constant : Constant  Value=0
  Subsystem : Subsystem
  Switch : Switch  Criteria=u2 > Threshold
  Out1 : Outport  VectorParamsAs1DForOutWhenUnconnected=off
  wires:
  Subsystem/1(Out1) -> Switch/3
  In1/1 -> Switch/1
  Switch/1 -> Out1/1
  Constant/1 -> Switch/2

== system Autopilot_q_full_5may_new/INITIALISE_PARAMS/If Action Subsystem/Structure_data_pert/Subsystem5 ==
  In1 : Inport
  Constant : Constant  Value=0
  Subsystem : Subsystem
  Switch : Switch  Criteria=u2 > Threshold
  Out1 : Outport  VectorParamsAs1DForOutWhenUnconnected=off
  wires:
  Constant/1 -> Switch/2
  Switch/1 -> Out1/1
  In1/1 -> Switch/1
  Subsystem/1(Out1) -> Switch/3

== system Autopilot_q_full_5may_new/INITIALISE_PARAMS/If Action Subsystem/Wind_data_pert/Subsystem1 ==
  In1 : Inport
  Constant : Constant  Value=0
  Subsystem : Subsystem
  Switch : Switch  Criteria=u2 > Threshold
  Out1 : Outport  VectorParamsAs1DForOutWhenUnconnected=off
  wires:
  Subsystem/1(Out1) -> Switch/3
  In1/1 -> Switch/1
  Switch/1 -> Out1/1
  Constant/1 -> Switch/2

== system Autopilot_q_full_5may_new/AUTOPILOT /Autopilot Transition mode/Forward transition/Pitch Controller/alpha controller ==
  acc_d : Inport
  Plane_state : Inport  Port=2
  Action Port : ActionPort  ActionPortLabel=if { }
  Aero_coffecients read2 : DataStoreRead  DataStoreName=Aero_cofficients  DataStoreElements=Aero_cofficients(:,:)
  Constant{6..11} (6 alike) : Constant
  Data Store Read : DataStoreRead  DataStoreName=Thrust_data_store  DataStoreElements=Thrust_data_store(:,:)
  Data Store Read1 : DataStoreRead  DataStoreName=Wind_data  DataStoreElements=Wind_data(:)
  Data Store Read13 : DataStoreRead  DataStoreName=propulsion_model  DataStoreElements=propulsion_model(:)
  Data Store Read15 : DataStoreRead  DataStoreName=Atmospheric_model
  Gain : Gain  Gain=57.3
  Gain1 : Gain  Gain=57.3
  MATLAB Function3 : MATLAB Function  TreatAsAtomicUnit=on
  PID Controller (2DOF)2 : simulink/Continuous/PID Controller (2DOF)  Controller=PID  TimeDomain=Discrete-time  SampleTime=0.01  IntegratorMethod=Forward Euler  FilterMethod=Forward Euler  Form=Parallel  UseFilter=on  ControllerParametersSource=internal  P=4.0  I=0.3  D=0.0  N=100  b=1  c=1  InitialConditionSource=internal  InitialConditionForIntegrator=0  InitialConditionForFilter=0  ExternalReset=none  ZeroCross=off  LimitOutput=off  UpperSaturationLimit=inf  LowerSaturationLimit=-inf  LinearizeAsGain=on  AntiWindupMode=none  Kb=1  TrackingMode=off  Kt=1  PParamMin=[]  PParamMax=[]  IParamMin=[]  IParamMax=[]  DParamMin=[]  DParamMax=[]  NParamMin=[]  NParamMax=[]  bParamMin=[]  bParamMax=[]  cParamMin=[]  cParamMax=[]  KbParamMin=[]  KbParamMax=[]  KtParamMin=[]  KtParamMax=[]  POutMin=[]  POutMax=[]  IOutMin=[]  IOutMax=[]  DOutMin=[]  DOutMax=[]  NOutMin=[]  NOutMax=[]  bOutMin=[]  bOutMax=[]  cOutMin=[]  cOutMax=[]  KbOutMin=[]  KbOutMax=[]  KtOutMin=[]  KtOutMax=[]  IntegratorOutMin=[]  IntegratorOutMax=[]  FilterOutMin=[]  FilterOutMax=[]  SumOutMin=[]  SumOutMax=[]  Sum1OutMin=[]  Sum1OutMax=[]  Sum2OutMin=[]  Sum2OutMax=[]  Sum3OutMin=[]  Sum3OutMax=[]  SumI1OutMin=[]  SumI1OutMax=[]  SumI2OutMin=[]  SumI2OutMax=[]  SumI3OutMin=[]  SumI3OutMax=[]  SumDOutMin=[]  SumDOutMax=[]  SaturationOutMin=[]  SaturationOutMax=[]  IntegratorContinuousStateAttributes=''  IntegratorStateMustResolveToSignalObject=off  IntegratorRTWStateStorageClass=Auto  FilterContinuousStateAttributes=''  FilterStateMustResolveToSignalObject=off  FilterRTWStateStorageClass=Auto  DifferentiatorICPrevScaledInput=0  DifferentiatorOutMin=[]  DifferentiatorOutMax=[]  FilterDiffOutCoefMin=[]  FilterDiffOutCoefMax=[]  SumDenOutMin=[]  SumDenOutMax=[]  SumNumOutMin=[]  SumNumOutMax=[]  ReciprocalOutMin=[]  ReciprocalOutMax=[]  DivideOutMin=[]  DivideOutMax=[]  TunerSelectOption=Transfer Function Based (PID Tuner App)
  Scope : Scope  NumInputPorts=2
  Structure_data_read1 : DataStoreRead  DataStoreName=Structural_data  DataStoreElements=Structural_data(:,:)
  alpha : Trigonometry  Operator=atan2
  u : DataStoreRead  DataStoreName=Plane_state_store  DataStoreElements=Plane_state_store(1,1)
  w : DataStoreRead  DataStoreName=Plane_state_store  DataStoreElements=Plane_state_store(1,3)
  Output : Outport  VectorParamsAs1DForOutWhenUnconnected=off
  wires:
  PID Controller (2DOF)2/1 -> Output/1
  Plane_state/1 -> MATLAB Function3/2(Plane_state)
  acc_d/1 -> MATLAB Function3/1(acc_d)
  MATLAB Function3/1(alpha_d) -> Gain/1, PID Controller (2DOF)2/1
  w/1 -> alpha/1
  u/1 -> alpha/2
  alpha/1 -> Gain1/1, PID Controller (2DOF)2/2
  Data Store Read/1 -> MATLAB Function3/5(Thrust)
  Aero_coffecients read2/1 -> MATLAB Function3/3(aero_data)
  Structure_data_read1/1 -> MATLAB Function3/4(structure_data)
  Gain1/1 -> Scope/2
  Gain/1 -> Scope/1
  Data Store Read1/1 -> MATLAB Function3/6(Wind_ned)
  Data Store Read13/1 -> MATLAB Function3/7(propulsion_data)
  Data Store Read15/1 -> MATLAB Function3/8(atmos_data)
  Constant6/1 -> MATLAB Function3/9(data2)
  Constant7/1 -> MATLAB Function3/10(data3)
  Constant8/1 -> MATLAB Function3/11(data4)
  Constant9/1 -> MATLAB Function3/12(data5)
  Constant10/1 -> MATLAB Function3/13(data6)
  Constant11/1 -> MATLAB Function3/14(data7)

== system Autopilot_q_full_5may_new/AUTOPILOT /Autopilot Transition mode/Forward transition/Pitch Controller/theta controller ==
  time : Inport
  a_x_d : Inport  Port=2
  alpha_trim : Inport  Port=3
  Action Port : ActionPort  ActionPortLabel=else { }
  Data Store Read1 : DataStoreRead  DataStoreName=Thrust_data_store  DataStoreElements=Thrust_data_store(1,1:8)
  Gain : Gain  Gain=57.3
  Gain1 : Gain  Gain=57.3
  MATLAB Function3 : MATLAB Function  TreatAsAtomicUnit=on
  PID Controller (2DOF)2 : simulink/Continuous/PID Controller (2DOF)  Controller=PID  TimeDomain=Discrete-time  SampleTime=0.01  IntegratorMethod=Forward Euler  FilterMethod=Forward Euler  Form=Parallel  UseFilter=on  ControllerParametersSource=internal  P=4.0  I=0.0  D=0  N=100  b=1  c=1  InitialConditionSource=internal  InitialConditionForIntegrator=0  InitialConditionForFilter=0  ExternalReset=none  LimitOutput=off  UpperSaturationLimit=inf  LowerSaturationLimit=-inf  LinearizeAsGain=on  AntiWindupMode=none  Kb=1  TrackingMode=off  Kt=1  PParamMin=[]  PParamMax=[]  IParamMin=[]  IParamMax=[]  DParamMin=[]  DParamMax=[]  NParamMin=[]  NParamMax=[]  bParamMin=[]  bParamMax=[]  cParamMin=[]  cParamMax=[]  KbParamMin=[]  KbParamMax=[]  KtParamMin=[]  KtParamMax=[]  POutMin=[]  POutMax=[]  IOutMin=[]  IOutMax=[]  DOutMin=[]  DOutMax=[]  NOutMin=[]  NOutMax=[]  bOutMin=[]  bOutMax=[]  cOutMin=[]  cOutMax=[]  KbOutMin=[]  KbOutMax=[]  KtOutMin=[]  KtOutMax=[]  IntegratorOutMin=[]  IntegratorOutMax=[]  FilterOutMin=[]  FilterOutMax=[]  SumOutMin=[]  SumOutMax=[]  Sum1OutMin=[]  Sum1OutMax=[]  Sum2OutMin=[]  Sum2OutMax=[]  Sum3OutMin=[]  Sum3OutMax=[]  SumI1OutMin=[]  SumI1OutMax=[]  SumI2OutMin=[]  SumI2OutMax=[]  SumI3OutMin=[]  SumI3OutMax=[]  SumDOutMin=[]  SumDOutMax=[]  SaturationOutMin=[]  SaturationOutMax=[]  IntegratorContinuousStateAttributes=''  IntegratorStateMustResolveToSignalObject=off  IntegratorRTWStateStorageClass=Auto  FilterContinuousStateAttributes=''  FilterStateMustResolveToSignalObject=off  FilterRTWStateStorageClass=Auto  DifferentiatorICPrevScaledInput=0  DifferentiatorOutMin=[]  DifferentiatorOutMax=[]  FilterDiffOutCoefMin=[]  FilterDiffOutCoefMax=[]  SumDenOutMin=[]  SumDenOutMax=[]  SumNumOutMin=[]  SumNumOutMax=[]  ReciprocalOutMin=[]  ReciprocalOutMax=[]  DivideOutMin=[]  DivideOutMax=[]  TunerSelectOption=Transfer Function Based (PID Tuner App)
  Scope : Scope  NumInputPorts=2
  mass : DataStoreRead  DataStoreName=Structural_data  DataStoreElements=Structural_data(1,1)
  theta : DataStoreRead  DataStoreName=Plane_state_store  DataStoreElements=Plane_state_store(1,8)
  theta_dot : Outport  VectorParamsAs1DForOutWhenUnconnected=off
  wires:
  theta/1 -> PID Controller (2DOF)2/2, Gain1/1
  time/1 -> MATLAB Function3/1(t)
  Data Store Read1/1 -> MATLAB Function3/2(TT)
  a_x_d/1 -> MATLAB Function3/4(a_x_d)
  PID Controller (2DOF)2/1 -> theta_dot/1
  alpha_trim/1 -> MATLAB Function3/5(data)
  mass/1 -> MATLAB Function3/3(mass)
  MATLAB Function3/1(theta_d) -> Gain/1, PID Controller (2DOF)2/1
  Gain1/1 -> Scope/2
  Gain/1 -> Scope/1
